simulink model "dcmotor_simulation"  (R2021b)
settings: Solver=VariableStepAuto  StartTime=0.0  StopTime=6  RelTol=1e-3
values from neighbouring files (symbols this model uses):
  Bm = 0.03    [dcmotor_parameters.m]
  Jm = 0.02    [dcmotor_parameters.m]
  Ke = 0.02    [dcmotor_parameters.m]
  La = 0.1    [dcmotor_parameters.m]
  Ra = 0.01    [dcmotor_parameters.m]
  TL = 0    [dcmotor_parameters.m]
  Va = 12    [dcmotor_parameters.m]
libraries: simulink_extras x2, SignalEditorBlockLib x1
settings Model: Creator=sacka  LastModifiedBy=sacka

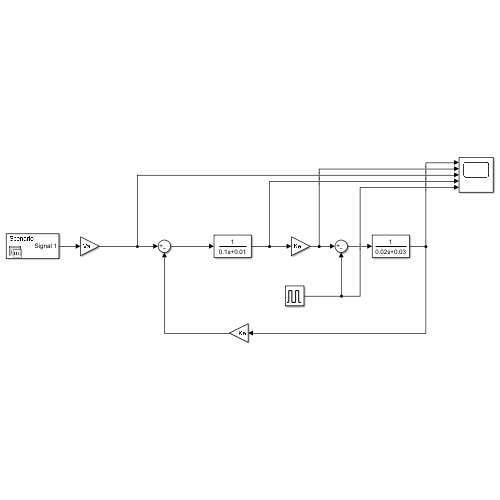
[thumbnail: Simulink's stored preview of the top-level diagram]
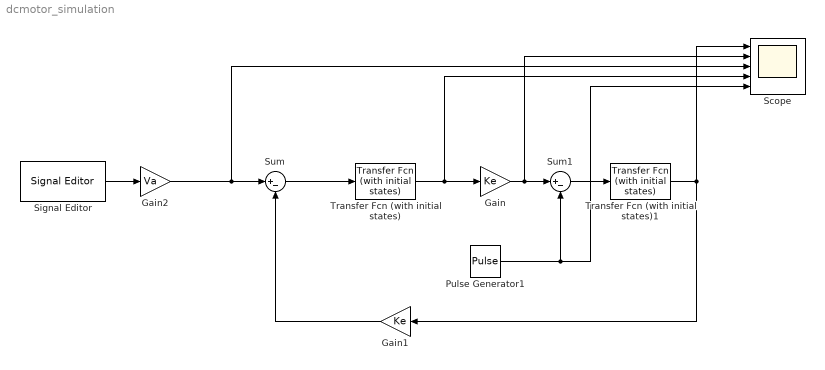
== system dcmotor_simulation ==
  Gain : Gain  Gain=Ke
  Gain1 : Gain  Gain=Ke
  Gain2 : Gain  Gain=Va
  Pulse Generator1 : DiscretePulseGenerator  PulseType=Time based  Amplitude=TL  Period=30  PulseWidth=90  PhaseDelay=6
  Scope : Scope  NumInputPorts=5
  Signal Editor : SignalEditorBlockLib/Signal Editor  FileName=dcmotor_signal_Va.mat  ActiveScenario=Scenario  ActiveSignal=Signal 1  IsBus=off  OutputBusObjectStr=Bus: BusObject  SampleTime=0  ZeroCross=off  OutputAfterFinalValue=Setting to zero  Unit=inherit  PreserveSignalName=on
  Sum : Sum  Inputs=|+-
  Sum1 : Sum  Inputs=|+-
  Transfer Fcn (with initial states) : simulink_extras/Additional Linear/Transfer Fcn (with initial states)  N=[1]  D=[La Ra]  X0=0
  Transfer Fcn (with initial states)1 : simulink_extras/Additional Linear/Transfer Fcn (with initial states)  N=[1]  D="[Jm  Bm]"  X0=0
  wires:
  Signal Editor/1 -> Gain2/1
  Sum/1 -> Transfer Fcn (with initial states)/1
  Gain/1 -> Scope/2, Sum1/1
  Sum1/1 -> Transfer Fcn (with initial states)1/1
  Transfer Fcn (with initial states)1/1 -> Scope/1, Gain1/1
  Gain1/1 -> Sum/2
  Transfer Fcn (with initial states)/1 -> Scope/4, Gain/1
  Pulse Generator1/1 -> Scope/5, Sum1/2
  Gain2/1 -> Scope/3, Sum/1
